simulink model "E2026_lateral_controler"  (R2023a)
settings: Solver=VariableStepAuto  StartTime=0.0  StopTime=10.0  RelTol=1e-3
libraries: drivingvehiclecontroller x1
settings Model: DataDictionary=modelo_bike_r23a.sldd  Creator=thailon  LastModifiedBy=thailon

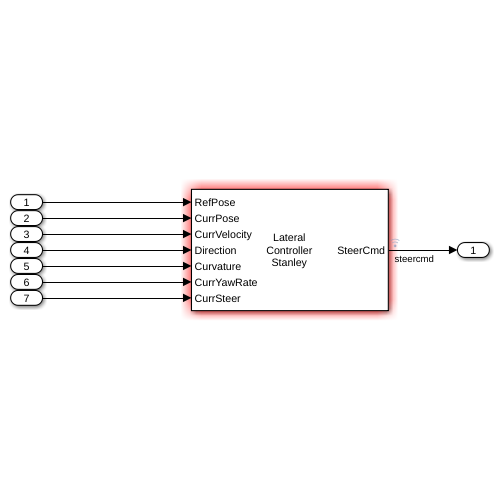
[thumbnail: Simulink's stored preview of the top-level diagram]
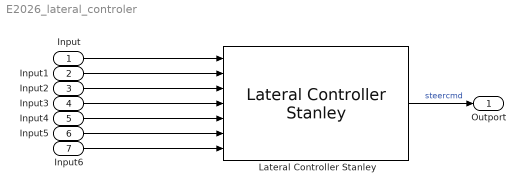
== system E2026_lateral_controler ==
  Input : Inport
  Input1 : Inport  Port=2
  Input2 : Inport  Port=3
  Input3 : Inport  Port=4
  Input4 : Inport  Port=5
  Input5 : Inport  Port=6
  Input6 : Inport  Port=7
  Lateral Controller Stanley : drivingvehiclecontroller/Lateral Controller Stanley  RequirementInfo="{}  %GIDa_64b493f0_f960_4d7a_b3c4_acd3e980d8ac"  ModelType=Dynamic bicycle model  PositionGainF=stanley_kpfw  PositionGainR=5  YawRateGain=ganho_yaw_rate  DelayGain=ganho_steering  VehicleMass=massa  Lf=distancia_eixo_frontal_centro_massa  Lr=distancia_eixo_ftraseiro_centro_massa  TireStiffness=rigidez_lateral_pneu_frontal  Wheelbase=wheelbase  MaxSteeringAngle=max_steering_angle
  Outport : Outport
  wires:
  Lateral Controller Stanley/1 -> Outport/1  "steercmd"
  Input/1 -> Lateral Controller Stanley/1
  Input1/1 -> Lateral Controller Stanley/2
  Input2/1 -> Lateral Controller Stanley/3
  Input3/1 -> Lateral Controller Stanley/4
  Input4/1 -> Lateral Controller Stanley/5
  Input5/1 -> Lateral Controller Stanley/6
  Input6/1 -> Lateral Controller Stanley/7
